simulink library "mbed_lib_hk"  (R2015a)
settings: Solver=ode45  SolverMode=SingleTasking  StartTime=0.0  StopTime=10.0  RelTol=1e-3
undefined symbols (not defined in the file): A
libraries: mbed_lib x1
(part 2 of 2)

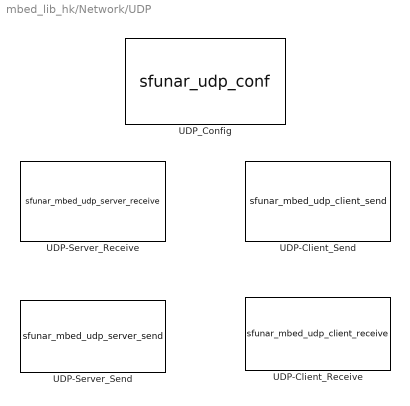
== system mbed_lib_hk/Network/UDP ==
  UDP-Client_Receive : S-Function  FunctionName=sfunar_mbed_udp_client_receive  Parameters=sock_ID, caOutputPorts, SampleTime  mask{sock_ID=2, caOutputPorts={'uint8' 'uint16'}, SampleTime=0}
      mask prompts: sock_ID "Socket ID:"; caOutputPorts "Output port data types (cell array):"; SampleTime "Sample time (-1 for inherited):"
      mask init:
      | sock_ID = get_param(gcbh,'sock_ID');
      | MaskDisplay = ['disp(''UDP-Client\nReceive\nId: ' num2str(sock_ID) ''');'];
      | set_param(gcb, 'MaskDisplay', MaskDisplay);
      mask TypeOptions sock_ID: 1 | 2 | 3 | 4 | 5 | 6 | 7 | 8
      mask Display: disp('UDP-Client\nReceive\nId: 2');
  UDP-Client_Send : S-Function  FunctionName=sfunar_mbed_udp_client_send  Parameters=sock_ID, des_IP, des_port, caInputPorts, SampleTime, nBufferBytes  mask{sock_ID=2, des_IP='192.168.0.50', des_port=5001, caInputPorts={'uint8' 'uint32' 'uint16'}, SampleTime=0, nBufferBytes=0}
      mask prompts: sock_ID "Socket ID:"; des_IP "Destination IP address:"; des_port "Destination Port:"; caInputPorts "Input port (unpacked) data types (cell array):"; SampleTime "Sample time (-1 for inherited):"
      mask init:
      | desip = get_param(gcbh,'des_ip');
      | desp = get_param(gcbh,'des_port');
      | sock_ID = get_param(gcbh,'sock_ID');
      | MaskDisplay = ['disp(''UDP-Client\nSend\nId: ' num2str(sock_ID)...
      |                 '\n Dest.: ' desip(2:end-1) ':' desp ''');'];
      | set_param(gcb, 'MaskDisplay', MaskDisplay);
      mask TypeOptions sock_ID: 1 | 2 | 3 | 4 | 5 | 6 | 7 | 8
      mask Display: disp('UDP-Client\nSend\nId: 2\n Dest.: 192.168.0.50:5001');
  UDP-Server_Receive : S-Function  FunctionName=sfunar_mbed_udp_server_receive  Parameters=sock_ID, src_port, caOutputPorts, SampleTime  mask{sock_ID=1, src_port=5001, caOutputPorts={'uint8' 'uint16' 'uint32'}, SampleTime=0}
      mask prompts: sock_ID "Socket ID:"; src_port "Source Port:"; caOutputPorts "Output port data types (cell array):"; SampleTime "Sample time (-1 for inherited):"
      mask init:
      | desp = get_param(gcbh,'src_port');
      | sock_ID = get_param(gcbh,'sock_ID');
      | MaskDisplay = ['disp(''UDP-Server\nReceive\nId: ' num2str(sock_ID)...
      |                 '\nSrv.- Port: ' desp ''');'];
      | set_param(gcb, 'MaskDisplay', MaskDisplay);
      mask TypeOptions sock_ID: 1 | 2 | 3 | 4 | 5 | 6 | 7 | 8
      mask Display: disp('UDP-Server\nReceive\nId: 1\nSrv.- Port: 5001');
  UDP-Server_Send : S-Function  FunctionName=sfunar_mbed_udp_server_send  Parameters=sock_ID, des_IP, srv_port, caInputPorts, SampleTime, nBufferBytes  mask{sock_ID=1, des_IP=0, srv_port=5002, caInputPorts={'uint8' 'uint16' 'uint32'}, SampleTime=0, nBufferBytes=0}
      mask prompts: sock_ID "Socket ID:"; des_IP "Destination IP address:"; srv_port "Destination Port:"; caInputPorts "Input port (unpacked) data types (cell array):"; SampleTime "Sample time (-1 for inherited):"
      mask init:
      | %desip = get_param(gcbh,'des_ip');
      | desp = get_param(gcbh,'srv_port');
      | sock_ID = get_param(gcbh,'sock_ID');
      | MaskDisplay = ['disp(''UDP-Server\nSend\nId: ' num2str(sock_ID) ''');'];
      | set_param(gcb, 'MaskDisplay', MaskDisplay);
      mask TypeOptions sock_ID: 1 | 2 | 3 | 4 | 5 | 6 | 7 | 8
      mask Display: disp('UDP-Server\nSend\nId: 1');
  UDP_Config : S-Function  FunctionName=sfunar_udp_conf  Parameters=ip_addr, sub_mask, gateway  mask{ip_addr='127.0.0.1', sub_mask='255.255.255.0', gateway='0.0.0.0', SampleTime=-1, DEFAULT_UDP_RECVMBOX_SIZE=8, TCPIP_THREAD_STACKSIZE=1024, TCPIP_THREAD_PRIO=Normal, PBUF_POOL_SIZE=5, TCP_MSS=1460}
      mask prompts: ip_addr "IP-Address"; sub_mask "Sub-Netmask"; SampleTime "Sample time (-1 for inherited):"; DEFAULT_UDP_RECVMBOX_SIZE "UDP Receive M-Box size"; TCPIP_THREAD_STACKSIZE "TCP/IP Thread Stacksize"; TCPIP_THREAD_PRIO "TCP/IP Thread Prio"; PBUF_POOL_SIZE "PBuf Pool Size"; TCP_MSS "TCP Maximun Segment Size"
      mask init:
      | ip = get_param(gcbh,'ip_addr');
      | subm = get_param(gcbh,'sub_mask');
      | MaskDisplay = ['disp(''UDP\nConfiguration\nIP: ' ip(2:end-1) ...
      |                 '\nSub-M.: ' subm(2:end-1) ''');'];
      | set_param(gcbh, 'MaskDisplay', MaskDisplay);
      settings: CopyFcn=|
      | fid = fopen('lwipopts.h','r+t');
      | lwipopts = textscan(fid,'%s','delimiter','\n');
      settings: DestroyFcn=|
      | try
      | fclose(fid);
      | catch ME
      | end
      | disp('Destroy')
      mask Callback DEFAULT_UDP_RECVMBOX_SIZE:
      | try
      |   %'isempty' is much faster then @isempty
      | pos_ti_th_ss = find(~cellfun('isempty',strfind(lwipopts{1,1},'DEFAULT_UDP_RECVMBOX_SIZE')));
      | lwipopts{1,1}{pos_ti_th_ss(1)} = ...
      |     sprintf('#define DEFAULT_UDP_RECVMBOX_SIZE\t%d',...
      |             get_param(gcb,'TCPIP_THREAD_STACKSIZE'));
      | 
      | for row = 1:length(lwipopts{1,1})
      |   fprintf(fid, '%s\n', lwipopts{1,1}{row});
      | end
      | 
      | catch exeption
      | end
      mask Callback TCPIP_THREAD_STACKSIZE:
      | try
      | pos_ti_th_ss = find(~cellfun('isempty',strfind(lwipopts{1,1},'TCPIP_THREAD_STACKSIZE')));
      | lwipopts{1,1}{pos_ti_th_ss(1)} = ...
      |     sprintf('#define TCPIP_THREAD_STACKSIZE\t%d',...
      |             get_param(gcb,'TCPIP_THREAD_STACKSIZE'));
      | 
      | for row = 1:length(lwipopts{1,1})
      |   fprintf(fid, '%s\n', lwipopts{1,1}{row});
      | end
      | 
      | catch exeption
      | end
      mask TypeOptions TCPIP_THREAD_PRIO: Idle | Low | Below Normal | Normal | Above Normal | High | Realtime
      mask Callback PBUF_POOL_SIZE:
      | try
      | pos_ti_th_ss = find(~cellfun('isempty',strfind(lwipopts{1,1},'PBUF_POOL_SIZE')));
      | lwipopts{1,1}{pos_ti_th_ss(1)} = ...
      |     sprintf('#define PBUF_POOL_SIZE\t%d',...
      |             get_param(gcb,'TCPIP_THREAD_STACKSIZE'));
      | 
      | for row = 1:length(lwipopts{1,1})
      |   fprintf(fid, '%s\n', lwipopts{1,1}{row});
      | end
      | 
      | catch exeption
      | end
      mask Callback TCP_MSS:
      | try
      | pos_ti_th_ss = find(~cellfun('isempty',strfind(lwipopts{1,1},'TCP_MSS')));
      | lwipopts{1,1}{pos_ti_th_ss(1)} = ...
      |     sprintf('#define TCP_MSS\t%d',...
      |             get_param(gcb,'TCPIP_THREAD_STACKSIZE'));
      | 
      | for row = 1:length(lwipopts{1,1})
      |   fprintf(fid, '%s\n', lwipopts{1,1}{row});
      | end
      | 
      | catch exeption
      | end
      mask Display: disp('UDP\nConfiguration\nIP: 127.0.0.1\nSub-M.: 255.255.255.0');

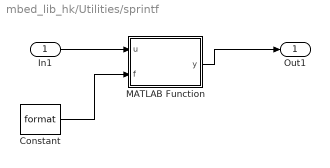
== system mbed_lib_hk/Utilities/sprintf ==
  In1 : Inport
  Constant : Constant  Value=format
  MATLAB Function : MATLAB Function  TreatAsAtomicUnit=on
  Out1 : Outport
  wires:
  In1/1 -> MATLAB Function/1(u)
  MATLAB Function/1(y) -> Out1/1
  Constant/1 -> MATLAB Function/2(f)

== matlab function mbed_lib_hk/Utilities/sprintf/MATLAB Function ==
  data: u input; y output; f input
function y = fcn(u,f)
buffer = char(zeros(1,15));
% geht mit 2012b noch nicht aber mit 2014a oder 2013: coder.cinclude('stdio.h');
coder.ceval('#ifdef _WIN32 //');
  if f == 1
    coder.ceval('_snprintf', coder.ref(buffer(int32(1))),int32(size(buffer,2)), ['%f' char(13) char(10) 0], u);
  elseif f == 2
    coder.ceval('_snprintf', coder.ref(buffer(int32(1))),int32(size(buffer,2)), ['%d' char(13) char(10) 0], u);
  elseif f == 3
    coder.ceval('_snprintf', coder.ref(buffer(int32(1))),int32(size(buffer,2)), ['%f' 0], u);
  elseif f == 4
    coder.ceval('_snprintf', coder.ref(buffer(int32(1))),int32(size(buffer,2)), ['%d' 0], u);
  end
coder.ceval('#else //');
  if f == 1
    coder.ceval('snprintf', coder.ref(buffer(int32(1))),int32(size(buffer,2)), ['%f' char(13) char(10) 0], u);
  elseif f == 2
    coder.ceval('snprintf', coder.ref(buffer(int32(1))),int32(size(buffer,2)), ['%d' char(13) char(10) 0], u);
  elseif f == 3
    coder.ceval('snprintf', coder.ref(buffer(int32(1))),int32(size(buffer,2)), ['%f' 0], u);
  elseif f == 4
    coder.ceval('snprintf', coder.ref(buffer(int32(1))),int32(size(buffer,2)), ['%d' 0], u);
  end
coder.ceval('#endif //');
y = uint8(buffer);
